simulink model "lab1_system3"  (R2024a)
settings: Solver=VariableStepAuto  StartTime=0.0  StopTime=10.0  RelTol=1e-3
undefined symbols (not defined in the file): a0, a1, a2, b0, b1, b2
settings Model: Creator=alexivanov  LastModifiedBy=alexivanov

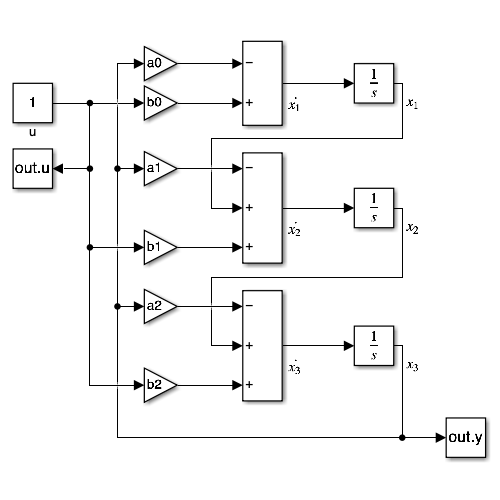
[thumbnail: Simulink's stored preview of the top-level diagram]
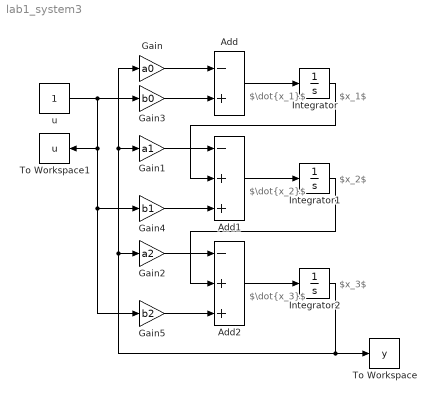
== system lab1_system3 ==
  note: $\dot{x_1}$
  note: $x_1$
  note: $\dot{x_2}$
  note: $x_2$
  note: $\dot{x_3}$
  note: $x_3$
  Add : Sum  Inputs=-+
  Add1 : Sum  Inputs=-++
  Add2 : Sum  Inputs=-++
  Gain : Gain  Gain=a0
  Gain1 : Gain  Gain=a1
  Gain2 : Gain  Gain=a2
  Gain3 : Gain  Gain=b0
  Gain4 : Gain  Gain=b1
  Gain5 : Gain  Gain=b2
  Integrator : Integrator
  Integrator1 : Integrator
  Integrator2 : Integrator
  To Workspace : ToWorkspace  VariableName=y  SaveFormat=Timeseries  SampleTime=-1
  To Workspace1 : ToWorkspace  VariableName=u  SaveFormat=Timeseries  SampleTime=-1
  u : Constant  SampleTime=0
  wires:
  Gain3/1 -> Add/2
  u/1 -> To Workspace1/1, Gain5/1, Gain4/1, Gain3/1
  Gain/1 -> Add/1
  Add/1 -> Integrator/1
  Gain1/1 -> Add1/1
  Integrator/1 -> Add1/2
  Gain4/1 -> Add1/3
  Add1/1 -> Integrator1/1
  Gain2/1 -> Add2/1
  Integrator1/1 -> Add2/2
  Gain5/1 -> Add2/3
  Add2/1 -> Integrator2/1
  Integrator2/1 -> Gain/1, Gain1/1, Gain2/1, To Workspace/1
